simulink model "bldc_model"  (R2014b)
settings: Solver=ode3  StartTime=0.0  StopTime=tdur  FixedStep=dt  RelTol=1e-3
values from neighbouring files (symbols this model uses):
  dt = CONST.dt    [bldc_discrete_current.m]    (also in bldc_discrete_speed.m; bldc_discrete_torque.m; bldc_model_basic.m = 1e-06; bldc_model_run.m = 1e-05)
  theta_m_0 = 0    [bldc_model_run.m]
  w_m_0 = 4000*rpm2rps    [bldc_model_run.m]
libraries: simulink x1, tool x1
settings Model: Creator=root  LastModifiedBy=root
settings DebuggingCC: FrameProcessingCompatibilityMsg=error

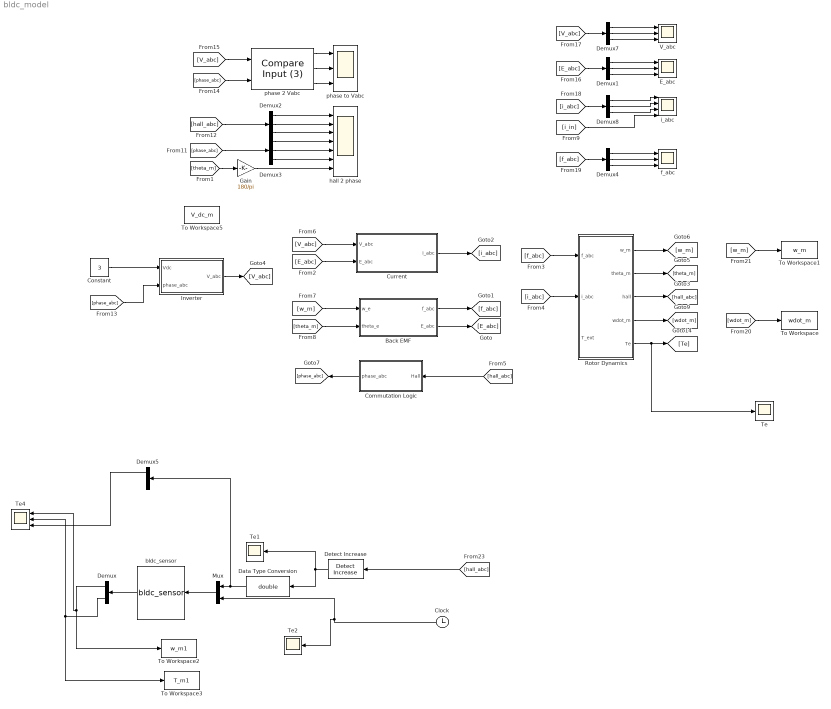
== system bldc_model ==
  Back EMF : Subsystem
  Clock : Clock
  Commutation Logic : Subsystem
  Constant : Constant  Value=3
  Current : Subsystem
  Data Type Conversion : DataTypeConversion  OutDataTypeStr=double  SampleTime=dt
  Demux : Demux  Outputs=2
  Demux{1..5,7..8} (7 alike) : Demux  Outputs=3
  Detect Increase : simulink/Logic and Bit Operations/Detect Increase  vinit=0.0  InputProcessing=Inherited  OutDataTypeStr=uint8
  E_abc : Scope  NumInputPorts=3
      settings: TimeRange=60  YMin=18000~-5~-5  YMax=20500~5~5  SaveName=ScopeData6
  Gain : Gain  Gain=180/pi
  Inverter : Subsystem
  Mux : Mux  Inputs=2
  Rotor Dynamics : Subsystem
  Te : Scope
      settings: TimeRange=1  YMin=1.2e-05  YMax=2.4e-05  SaveName=ScopeData7
  Te1 : Scope
      settings: TimeRange=1  YMin=1.2e-05  YMax=2.4e-05  SampleInput=on
  Te2 : Scope
      settings: TimeRange=1  YMin=1.2e-05  YMax=2.4e-05  SaveName=ScopeData3  SampleInput=on
  Te4 : Scope  NumInputPorts=3
      settings: TimeRange=1  YMin=86.6~-4~-5  YMax=87.3~4~5  SaveName=ScopeData10  SampleInput=on  SampleTime=dt
  To Workspace : ToWorkspace  VariableName=wdot_m  SampleTime=-1
  To Workspace1 : ToWorkspace  VariableName=w_m  SampleTime=-1
  To Workspace2 : ToWorkspace  VariableName=w_m1  SampleTime=-1
  To Workspace3 : ToWorkspace  VariableName=T_m1  SampleTime=-1
  To Workspace5 : ToWorkspace  VariableName=V_dc_m  SampleTime=-1
  V_abc : Scope  NumInputPorts=3
      settings: TimeRange=60  YMin=18000~-5~-5  YMax=20500~5~5  SaveName=ScopeData5
  bldc_sensor : MATLABFcn  MATLABFcn=bldc_sensor  OutputDimensions=[2,1]  Output1D=off  SampleTime=dt
  f_abc : Scope  NumInputPorts=3
      settings: TimeRange=60  YMin=18000~-5~-5  YMax=20500~5~5
  hall 2 phase : Scope  NumInputPorts=7
      settings: TimeRange=5  YMin=0~0~0~-1~-1~-1~-200  YMax=1~1~1~1~1~1~200  SaveName=ScopeData8  SampleInput=on
  i_abc : Scope  NumInputPorts=4
      settings: TimeRange=60  YMin=18000~-5~-5~-5  YMax=20500~5~5~5  SaveName=ScopeData4  SampleInput=on
  phase 2 Vabc : tool/Compare Input (3)
  phase to Vabc : Scope  NumInputPorts=3
      settings: TimeRange=5  YMin=-1~-1~-1  YMax=1~1~1  SaveName=ScopeData2  SampleInput=on
  wires:
  [E_abc] -> Current/2(E_abc)
  Back EMF/2(E_abc) -> [E_abc]
  Back EMF/1(f_abc) -> [f_abc]
  [i_abc] -> Rotor Dynamics/2(i_abc)
  Rotor Dynamics/3(hall) -> [hall_abc]
  Commutation Logic/1(phase_abc) -> [phase_abc]
  [V_abc] -> Current/1(V_abc)
  Rotor Dynamics/2(theta_m) -> [theta_m]
  Rotor Dynamics/1(w_m) -> [w_m]
  [theta_m] -> Back EMF/2(theta_e)
  [w_m] -> Back EMF/1(w_e)
  Inverter/1(V_abc) -> [V_abc]
  Rotor Dynamics/4(wdot_m) -> [wdot_m]
  Demux1/3 -> E_abc/3
  Demux1/2 -> E_abc/2
  Demux1/1 -> E_abc/1
  Demux4/3 -> f_abc/3
  Demux4/2 -> f_abc/2
  Demux4/1 -> f_abc/1
  [f_abc] -> Rotor Dynamics/1(f_abc)
  phase 2 Vabc/3 -> phase to Vabc/3
  phase 2 Vabc/2 -> phase to Vabc/2
  phase 2 Vabc/1 -> phase to Vabc/1
  Current/1(i_abc) -> [i_abc]
  Demux2/3 -> hall 2 phase/3
  Demux2/2 -> hall 2 phase/2
  Demux2/1 -> hall 2 phase/1
  Demux3/2 -> hall 2 phase/5
  Demux3/1 -> hall 2 phase/4
  Demux3/3 -> hall 2 phase/6
  [theta_m] -> Gain/1
  [phase_abc] -> Demux3/1
  Gain/1 -> hall 2 phase/7
  [hall_abc] -> Demux2/1
  [phase_abc] -> Inverter/2(phase_abc)
  [phase_abc] -> phase 2 Vabc/2
  [E_abc] -> Demux1/1
  Demux7/3 -> V_abc/3
  Demux7/2 -> V_abc/2
  Demux7/1 -> V_abc/1
  [V_abc] -> Demux7/1
  Demux8/3 -> i_abc/3
  Demux8/2 -> i_abc/2
  Demux8/1 -> i_abc/1
  [i_abc] -> Demux8/1
  [f_abc] -> Demux4/1
  [wdot_m] -> To Workspace/1
  [w_m] -> To Workspace1/1
  [V_abc] -> phase 2 Vabc/1
  [hall_abc] -> Commutation Logic/1("Hall ")
  Detect Increase/1 -> Data Type Conversion/1, Te1/1
  Clock/1 -> Mux/2, Te2/1
  Data Type Conversion/1 -> Demux5/1, Mux/1
  Mux/1 -> bldc_sensor/1
  bldc_sensor/1 -> Demux/1
  Demux/1 -> To Workspace2/1, Te4/1
  Demux/2 -> To Workspace3/1, Te4/2
  [i_in] -> i_abc/4
  [hall_abc] -> Detect Increase/1
  Rotor Dynamics/5(Te) -> Te/1, [Te]
  Constant/1 -> Inverter/1(Vdc)
  Demux5/1 -> Te4/3

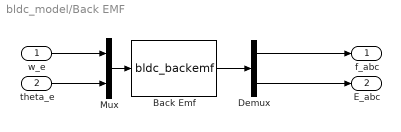
== system bldc_model/Back EMF ==
  w_e : Inport
  theta_e : Inport  Port=2
  Back Emf : MATLABFcn  MATLABFcn=bldc_backemf  OutputDimensions=[6,1]  Output1D=off
  Demux : Demux  Outputs=[3 3]
  Mux : Mux  Inputs=[1;1]
  f_abc : Outport
  E_abc : Outport  Port=2
  wires:
  Demux/2 -> E_abc/1
  Demux/1 -> f_abc/1
  w_e/1 -> Mux/1
  Back Emf/1 -> Demux/1
  Mux/1 -> Back Emf/1
  theta_e/1 -> Mux/2

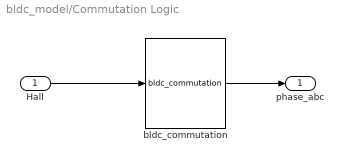
== system bldc_model/Commutation Logic ==
  "Hall " : Inport
  bldc_commutation : MATLABFcn  MATLABFcn=bldc_commutation  OutputDimensions=[3,1]  Output1D=off
  phase_abc : Outport
  wires:
  "Hall "/1 -> bldc_commutation/1
  bldc_commutation/1 -> phase_abc/1

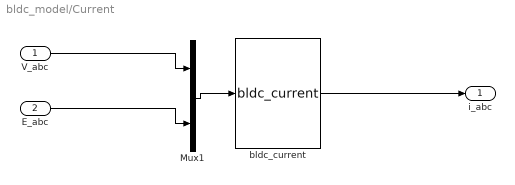
== system bldc_model/Current ==
  V_abc : Inport
  E_abc : Inport  Port=2
  Mux1 : Mux  Inputs=[3;3]
  bldc_current : MATLABFcn  MATLABFcn=bldc_current  OutputDimensions=[3,1]  Output1D=off
  i_abc : Outport
  wires:
  Mux1/1 -> bldc_current/1
  E_abc/1 -> Mux1/2
  V_abc/1 -> Mux1/1
  bldc_current/1 -> i_abc/1

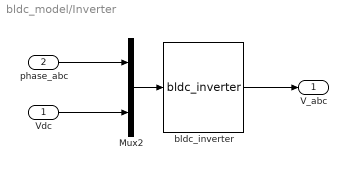
== system bldc_model/Inverter ==
  Vdc : Inport
  phase_abc : Inport  Port=2
  Mux2 : Mux  Inputs=[3;1]
  bldc_inverter : MATLABFcn  MATLABFcn=bldc_inverter  OutputDimensions=[3,1]  Output1D=off
  V_abc : Outport
  wires:
  phase_abc/1 -> Mux2/1
  Vdc/1 -> Mux2/2
  Mux2/1 -> bldc_inverter/1
  bldc_inverter/1 -> V_abc/1

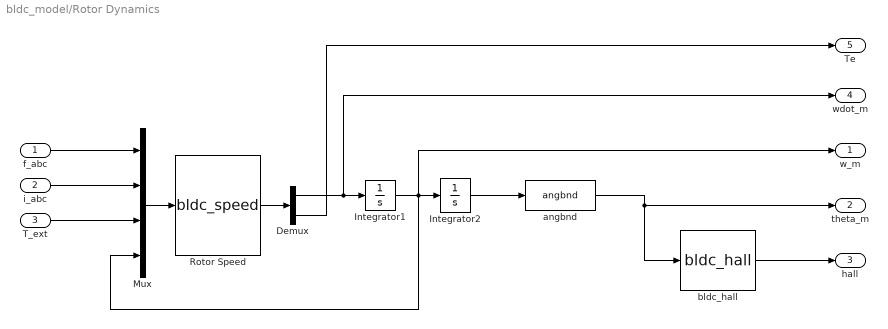
== system bldc_model/Rotor Dynamics ==
  f_abc : Inport
  i_abc : Inport  Port=2
  T_ext : Inport  Port=3
  Demux : Demux  Outputs=2
  Integrator1 : Integrator  InitialCondition=w_m_0
  Integrator2 : Integrator  InitialCondition=theta_m_0
  Mux : Mux  Inputs=[3;3;1;1]
  Rotor Speed : MATLABFcn  MATLABFcn=bldc_speed  OutputDimensions=[2,1]  Output1D=off
  angbnd : MATLABFcn  MATLABFcn=angbnd
  bldc_hall : MATLABFcn  MATLABFcn=bldc_hall  Output1D=off
  w_m : Outport
  theta_m : Outport  Port=2
  hall : Outport  Port=3
  wdot_m : Outport  Port=4
  Te : Outport  Port=5
  wires:
  Rotor Speed/1 -> Demux/1
  T_ext/1 -> Mux/3
  i_abc/1 -> Mux/2
  Mux/1 -> Rotor Speed/1
  f_abc/1 -> Mux/1
  bldc_hall/1 -> hall/1
  Integrator2/1 -> angbnd/1
  Integrator1/1 -> w_m/1, Mux/4, Integrator2/1
  angbnd/1 -> theta_m/1, bldc_hall/1
  Demux/1 -> Integrator1/1, wdot_m/1
  Demux/2 -> Te/1
